simulink model "DpfIntfc_Delivery"  (Simulink 8.2)
settings: Solver=FixedStepDiscrete  StartTime=0.0  StopTime=10.0  FixedStep=0.001  RelTol=1e-3
undefined symbols (not defined in the file): DiscIntNeverNeededParam
libraries: simulink x15, DpfIntfc_Lib x1
(part 2 of 2)

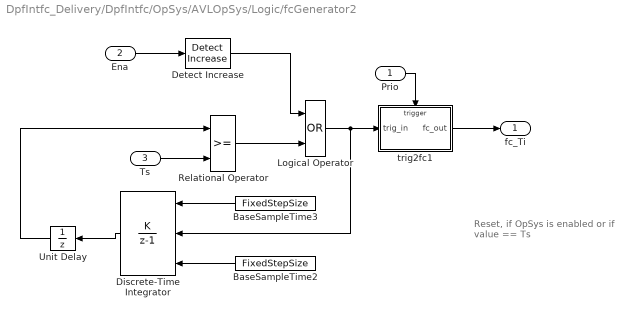
== system DpfIntfc_Delivery/DpfIntfc/OpSys/AVLOpSys/Logic/fcGenerator2 ==
  note: Reset, if OpSys is enabled or if value == Ts
  Prio : Inport
  Ena : Inport  Port=2
  Ts : Inport  Port=3
  BaseSampleTime2 : Constant  Value=FixedStepSize
  BaseSampleTime3 : Constant  Value=FixedStepSize
  Detect Increase : simulink/Logic and Bit Operations/Detect Increase  vinit=0.0  InputProcessing=Inherited  OutDataTypeStr=uint8
  Discrete-Time Integrator : DiscreteIntegrator  IntegratorMethod=Accumulation: Forward Euler  ExternalReset=rising  InitialConditionSource=external  SampleTime=-1  ICPrevOutput=DiscIntNeverNeededParam  ICPrevScaledInput=DiscIntNeverNeededParam
  Logical Operator : Logic  Operator=OR  AllPortsSameDT=off  OutDataTypeStr=boolean
  Relational Operator : RelationalOperator  OutDataTypeStr=boolean
  Unit Delay : UnitDelay  SampleTime=-1
  trig2fc1 : Subsystem
  fc_Ti : Outport
  wires:
  Unit Delay/1 -> Relational Operator/1
  Detect Increase/1 -> Logical Operator/1
  Logical Operator/1 -> Discrete-Time Integrator/2, trig2fc1/1(trig_in)
  Relational Operator/1 -> Logical Operator/2
  Ena/1 -> Detect Increase/1
  Discrete-Time Integrator/1 -> Unit Delay/1
  BaseSampleTime3/1 -> Discrete-Time Integrator/1
  BaseSampleTime2/1 -> Discrete-Time Integrator/3
  trig2fc1/1(fc_out) -> fc_Ti/1
  Prio/1 -> trig2fc1/Trigger
  Ts/1 -> Relational Operator/2

== system DpfIntfc_Delivery/DpfIntfc/OpSys/AVLOpSys/Logic/fcGenerator3 ==
  Prio : Inport
  Edge : Inport  Port=2
  Data Type Conversion : DataTypeConversion  OutDataTypeStr=boolean
  FixPt Relational Operator : RelationalOperator  Operator=>  OutDataTypeStr=boolean  ZeroCross=off
  Unit Delay : UnitDelay  SampleTime=-1
      settings: AttributesFormatString=SampleTime = %<SampleTime>\nInit = %<X0>
  trig2fc : Subsystem
  fc_RiseEdge : Outport
  wires:
  Unit Delay/1 -> FixPt Relational Operator/2
  Prio/1 -> trig2fc/Trigger
  trig2fc/1(fc_out) -> fc_RiseEdge/1
  Edge/1 -> Data Type Conversion/1
  Data Type Conversion/1 -> Unit Delay/1, FixPt Relational Operator/1
  FixPt Relational Operator/1 -> trig2fc/1(trig_in)

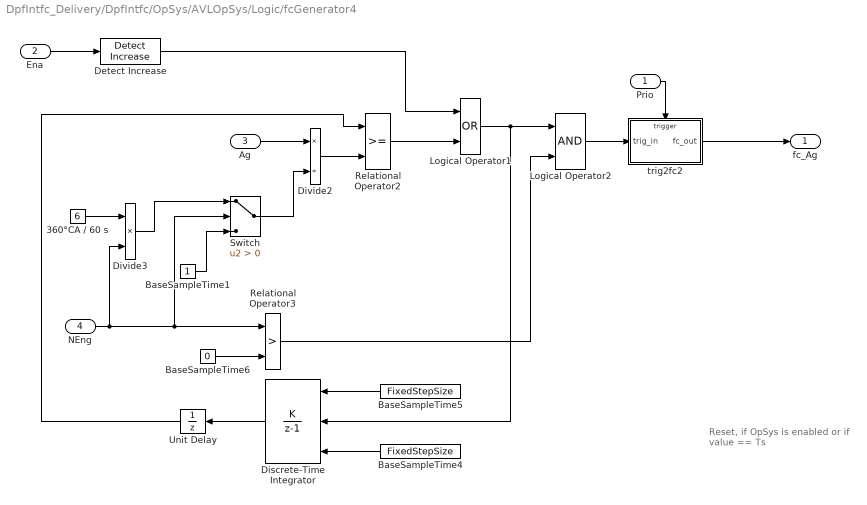
== system DpfIntfc_Delivery/DpfIntfc/OpSys/AVLOpSys/Logic/fcGenerator4 ==
  note: Reset, if OpSys is enabled or if value == Ts
  Prio : Inport
  Ena : Inport  Port=2
  Ag : Inport  Port=3
  NEng : Inport  Port=4
  360°CA / 60 s : Constant  Value=6
  BaseSampleTime1 : Constant
  BaseSampleTime4 : Constant  Value=FixedStepSize
  BaseSampleTime5 : Constant  Value=FixedStepSize
  BaseSampleTime6 : Constant  Value=0
  Detect Increase : simulink/Logic and Bit Operations/Detect Increase  vinit=0.0  InputProcessing=Inherited  OutDataTypeStr=uint8
  Discrete-Time Integrator : DiscreteIntegrator  IntegratorMethod=Accumulation: Forward Euler  ExternalReset=rising  InitialConditionSource=external  SampleTime=-1  ICPrevOutput=DiscIntNeverNeededParam  ICPrevScaledInput=DiscIntNeverNeededParam
  Divide2 : Product  Inputs=*/
  Divide3 : Product  Inputs=**
  Logical Operator1 : Logic  Operator=OR  AllPortsSameDT=off  OutDataTypeStr=boolean
  Logical Operator2 : Logic  AllPortsSameDT=off  OutDataTypeStr=boolean
  Relational Operator2 : RelationalOperator  OutDataTypeStr=boolean
  Relational Operator3 : RelationalOperator  Operator=>  OutDataTypeStr=boolean
  Switch : Switch  Criteria=u2 > Threshold
  Unit Delay : UnitDelay  SampleTime=-1
  trig2fc2 : Subsystem
  fc_Ag : Outport
  wires:
  BaseSampleTime1/1 -> Switch/3
  Switch/1 -> Divide2/2
  Divide3/1 -> Switch/1
  Unit Delay/1 -> Relational Operator2/1
  Relational Operator3/1 -> Logical Operator2/2
  Logical Operator2/1 -> trig2fc2/1(trig_in)
  Ag/1 -> Divide2/1
  Divide2/1 -> Relational Operator2/2
  360°CA / 60 s/1 -> Divide3/1
  BaseSampleTime6/1 -> Relational Operator3/2
  NEng/1 -> Divide3/2, Switch/2, Relational Operator3/1
  Logical Operator1/1 -> Discrete-Time Integrator/2, Logical Operator2/1
  Detect Increase/1 -> Logical Operator1/1
  Relational Operator2/1 -> Logical Operator1/2
  Ena/1 -> Detect Increase/1
  Discrete-Time Integrator/1 -> Unit Delay/1
  BaseSampleTime5/1 -> Discrete-Time Integrator/1
  BaseSampleTime4/1 -> Discrete-Time Integrator/3
  trig2fc2/1(fc_out) -> fc_Ag/1
  Prio/1 -> trig2fc2/Trigger

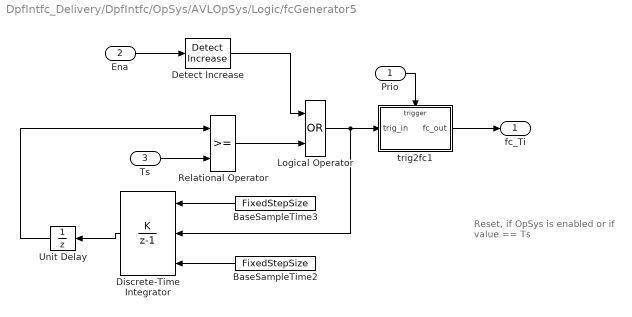
== system DpfIntfc_Delivery/DpfIntfc/OpSys/AVLOpSys/Logic/fcGenerator5 ==
  note: Reset, if OpSys is enabled or if value == Ts
  Prio : Inport
  Ena : Inport  Port=2
  Ts : Inport  Port=3
  BaseSampleTime2 : Constant  Value=FixedStepSize
  BaseSampleTime3 : Constant  Value=FixedStepSize
  Detect Increase : simulink/Logic and Bit Operations/Detect Increase  vinit=0.0  InputProcessing=Inherited  OutDataTypeStr=uint8
  Discrete-Time Integrator : DiscreteIntegrator  IntegratorMethod=Accumulation: Forward Euler  ExternalReset=rising  InitialConditionSource=external  SampleTime=-1  ICPrevOutput=DiscIntNeverNeededParam  ICPrevScaledInput=DiscIntNeverNeededParam
  Logical Operator : Logic  Operator=OR  AllPortsSameDT=off  OutDataTypeStr=boolean
  Relational Operator : RelationalOperator  OutDataTypeStr=boolean
  Unit Delay : UnitDelay  SampleTime=-1
  trig2fc1 : Subsystem
  fc_Ti : Outport
  wires:
  Unit Delay/1 -> Relational Operator/1
  Detect Increase/1 -> Logical Operator/1
  Logical Operator/1 -> Discrete-Time Integrator/2, trig2fc1/1(trig_in)
  Relational Operator/1 -> Logical Operator/2
  Ena/1 -> Detect Increase/1
  Discrete-Time Integrator/1 -> Unit Delay/1
  BaseSampleTime3/1 -> Discrete-Time Integrator/1
  BaseSampleTime2/1 -> Discrete-Time Integrator/3
  trig2fc1/1(fc_out) -> fc_Ti/1
  Prio/1 -> trig2fc1/Trigger
  Ts/1 -> Relational Operator/2

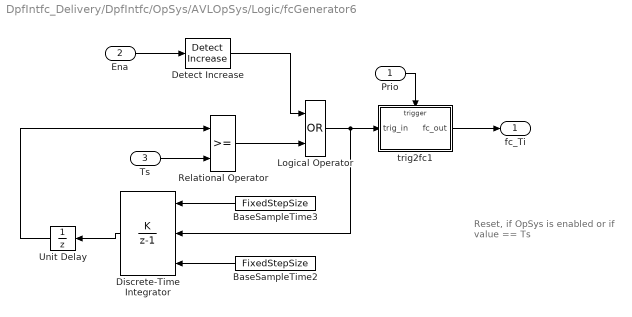
== system DpfIntfc_Delivery/DpfIntfc/OpSys/AVLOpSys/Logic/fcGenerator6 ==
  note: Reset, if OpSys is enabled or if value == Ts
  Prio : Inport
  Ena : Inport  Port=2
  Ts : Inport  Port=3
  BaseSampleTime2 : Constant  Value=FixedStepSize
  BaseSampleTime3 : Constant  Value=FixedStepSize
  Detect Increase : simulink/Logic and Bit Operations/Detect Increase  vinit=0.0  InputProcessing=Inherited  OutDataTypeStr=uint8
  Discrete-Time Integrator : DiscreteIntegrator  IntegratorMethod=Accumulation: Forward Euler  ExternalReset=rising  InitialConditionSource=external  SampleTime=-1  ICPrevOutput=DiscIntNeverNeededParam  ICPrevScaledInput=DiscIntNeverNeededParam
  Logical Operator : Logic  Operator=OR  AllPortsSameDT=off  OutDataTypeStr=boolean
  Relational Operator : RelationalOperator  OutDataTypeStr=boolean
  Unit Delay : UnitDelay  SampleTime=-1
  trig2fc1 : Subsystem
  fc_Ti : Outport
  wires:
  Unit Delay/1 -> Relational Operator/1
  Detect Increase/1 -> Logical Operator/1
  Logical Operator/1 -> Discrete-Time Integrator/2, trig2fc1/1(trig_in)
  Relational Operator/1 -> Logical Operator/2
  Ena/1 -> Detect Increase/1
  Discrete-Time Integrator/1 -> Unit Delay/1
  BaseSampleTime3/1 -> Discrete-Time Integrator/1
  BaseSampleTime2/1 -> Discrete-Time Integrator/3
  trig2fc1/1(fc_out) -> fc_Ti/1
  Prio/1 -> trig2fc1/Trigger
  Ts/1 -> Relational Operator/2

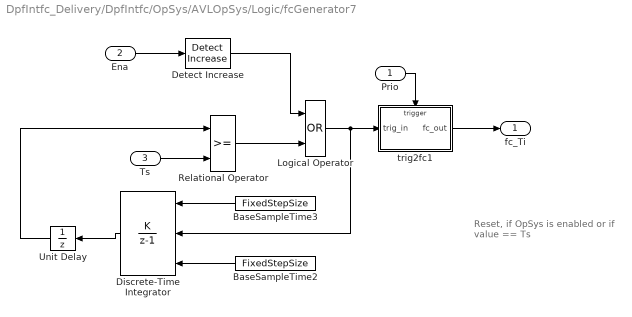
== system DpfIntfc_Delivery/DpfIntfc/OpSys/AVLOpSys/Logic/fcGenerator7 ==
  note: Reset, if OpSys is enabled or if value == Ts
  Prio : Inport
  Ena : Inport  Port=2
  Ts : Inport  Port=3
  BaseSampleTime2 : Constant  Value=FixedStepSize
  BaseSampleTime3 : Constant  Value=FixedStepSize
  Detect Increase : simulink/Logic and Bit Operations/Detect Increase  vinit=0.0  InputProcessing=Inherited  OutDataTypeStr=uint8
  Discrete-Time Integrator : DiscreteIntegrator  IntegratorMethod=Accumulation: Forward Euler  ExternalReset=rising  InitialConditionSource=external  SampleTime=-1  ICPrevOutput=DiscIntNeverNeededParam  ICPrevScaledInput=DiscIntNeverNeededParam
  Logical Operator : Logic  Operator=OR  AllPortsSameDT=off  OutDataTypeStr=boolean
  Relational Operator : RelationalOperator  OutDataTypeStr=boolean
  Unit Delay : UnitDelay  SampleTime=-1
  trig2fc1 : Subsystem
  fc_Ti : Outport
  wires:
  Unit Delay/1 -> Relational Operator/1
  Detect Increase/1 -> Logical Operator/1
  Logical Operator/1 -> Discrete-Time Integrator/2, trig2fc1/1(trig_in)
  Relational Operator/1 -> Logical Operator/2
  Ena/1 -> Detect Increase/1
  Discrete-Time Integrator/1 -> Unit Delay/1
  BaseSampleTime3/1 -> Discrete-Time Integrator/1
  BaseSampleTime2/1 -> Discrete-Time Integrator/3
  trig2fc1/1(fc_out) -> fc_Ti/1
  Prio/1 -> trig2fc1/Trigger
  Ts/1 -> Relational Operator/2

== system DpfIntfc_Delivery/DpfIntfc/OpSys/AVLOpSys/Logic/fcGenerator1/trig2fc1 ==
  trig_in : Inport
  fc : TriggerPort  TriggerType=function-call
  If Action Subsystem : Subsystem  TreatAsAtomicUnit=on
  fc_out : Outport
  wires:
  If Action Subsystem/1(fc) -> fc_out/1
  trig_in/1 -> If Action Subsystem/Enable

== system DpfIntfc_Delivery/DpfIntfc/OpSys/AVLOpSys/Logic/fcGenerator2/trig2fc1 ==
  trig_in : Inport
  fc : TriggerPort  TriggerType=function-call
  If Action Subsystem : Subsystem  TreatAsAtomicUnit=on
  fc_out : Outport
  wires:
  If Action Subsystem/1(fc) -> fc_out/1
  trig_in/1 -> If Action Subsystem/Enable

== system DpfIntfc_Delivery/DpfIntfc/OpSys/AVLOpSys/Logic/fcGenerator3/trig2fc ==
  trig_in : Inport
  fc : TriggerPort  TriggerType=function-call
  If Action Subsystem : Subsystem  TreatAsAtomicUnit=on
  fc_out : Outport
  wires:
  If Action Subsystem/1(fc) -> fc_out/1
  trig_in/1 -> If Action Subsystem/Enable

== system DpfIntfc_Delivery/DpfIntfc/OpSys/AVLOpSys/Logic/fcGenerator4/trig2fc2 ==
  trig_in : Inport
  fc : TriggerPort  TriggerType=function-call
  If Action Subsystem : Subsystem  TreatAsAtomicUnit=on
  fc_out : Outport
  wires:
  If Action Subsystem/1(fc) -> fc_out/1
  trig_in/1 -> If Action Subsystem/Enable

== system DpfIntfc_Delivery/DpfIntfc/OpSys/AVLOpSys/Logic/fcGenerator5/trig2fc1 ==
  trig_in : Inport
  fc : TriggerPort  TriggerType=function-call
  If Action Subsystem : Subsystem  TreatAsAtomicUnit=on
  fc_out : Outport
  wires:
  If Action Subsystem/1(fc) -> fc_out/1
  trig_in/1 -> If Action Subsystem/Enable

== system DpfIntfc_Delivery/DpfIntfc/OpSys/AVLOpSys/Logic/fcGenerator6/trig2fc1 ==
  trig_in : Inport
  fc : TriggerPort  TriggerType=function-call
  If Action Subsystem : Subsystem  TreatAsAtomicUnit=on
  fc_out : Outport
  wires:
  If Action Subsystem/1(fc) -> fc_out/1
  trig_in/1 -> If Action Subsystem/Enable

== system DpfIntfc_Delivery/DpfIntfc/OpSys/AVLOpSys/Logic/fcGenerator7/trig2fc1 ==
  trig_in : Inport
  fc : TriggerPort  TriggerType=function-call
  If Action Subsystem : Subsystem  TreatAsAtomicUnit=on
  fc_out : Outport
  wires:
  If Action Subsystem/1(fc) -> fc_out/1
  trig_in/1 -> If Action Subsystem/Enable

== system DpfIntfc_Delivery/DpfIntfc/OpSys/AVLOpSys/Logic/fcGenerator1/trig2fc1/If Action Subsystem ==
  Enable : EnablePort
  Function-Call Generator : simulink/Ports & Subsystems/Function-Call Generator  sample_time=-1  numberOfIterations=1
  fc : Outport
  wires:
  Function-Call Generator/1 -> fc/1

== system DpfIntfc_Delivery/DpfIntfc/OpSys/AVLOpSys/Logic/fcGenerator2/trig2fc1/If Action Subsystem ==
  Enable : EnablePort
  Function-Call Generator : simulink/Ports & Subsystems/Function-Call Generator  sample_time=-1  numberOfIterations=1
  fc : Outport
  wires:
  Function-Call Generator/1 -> fc/1

== system DpfIntfc_Delivery/DpfIntfc/OpSys/AVLOpSys/Logic/fcGenerator3/trig2fc/If Action Subsystem ==
  Enable : EnablePort
  Function-Call Generator : simulink/Ports & Subsystems/Function-Call Generator  sample_time=-1  numberOfIterations=1
  fc : Outport
  wires:
  Function-Call Generator/1 -> fc/1

== system DpfIntfc_Delivery/DpfIntfc/OpSys/AVLOpSys/Logic/fcGenerator4/trig2fc2/If Action Subsystem ==
  Enable : EnablePort
  Function-Call Generator : simulink/Ports & Subsystems/Function-Call Generator  sample_time=-1  numberOfIterations=1
  fc : Outport
  wires:
  Function-Call Generator/1 -> fc/1

== system DpfIntfc_Delivery/DpfIntfc/OpSys/AVLOpSys/Logic/fcGenerator5/trig2fc1/If Action Subsystem ==
  Enable : EnablePort
  Function-Call Generator : simulink/Ports & Subsystems/Function-Call Generator  sample_time=-1  numberOfIterations=1
  fc : Outport
  wires:
  Function-Call Generator/1 -> fc/1

== system DpfIntfc_Delivery/DpfIntfc/OpSys/AVLOpSys/Logic/fcGenerator6/trig2fc1/If Action Subsystem ==
  Enable : EnablePort
  Function-Call Generator : simulink/Ports & Subsystems/Function-Call Generator  sample_time=-1  numberOfIterations=1
  fc : Outport
  wires:
  Function-Call Generator/1 -> fc/1

== system DpfIntfc_Delivery/DpfIntfc/OpSys/AVLOpSys/Logic/fcGenerator7/trig2fc1/If Action Subsystem ==
  Enable : EnablePort
  Function-Call Generator : simulink/Ports & Subsystems/Function-Call Generator  sample_time=-1  numberOfIterations=1
  fc : Outport
  wires:
  Function-Call Generator/1 -> fc/1
